simulink model "Q_2_1_PID_with_Anti_Windup"  (R2024b)
settings: Solver=ode45  StartTime=0.0  StopTime=1  FixedStep=0.001  RelTol=1e-3
values from neighbouring files (symbols this model uses):
  delta_c = 1 / sqrt(2)    [PID_calculations.m]    (also in SS_Calculations.m)
  K_D = K_P * T_D    [PID_calculations.m]
  K_I = K_P / T_I    [PID_calculations.m]
  K_P = DeltaK * cos(DeltaPhi)    [PID_calculations.m]
  K_W = 1 / T_W    (= 1485.71428571)    [PID_calculations.m]
  T_L = 5 * w_gc    [PID_calculations.m]
  w_c = 2 * pi * 20    (= 125.663706144)    [PID_calculations.m]    (also in SS_Calculations.m = 314.159265359)
undefined symbols (not defined in the file or in its folder): gbox, rads2rpm, sens
settings Model: Creator=JS  LastModifiedBy=JS

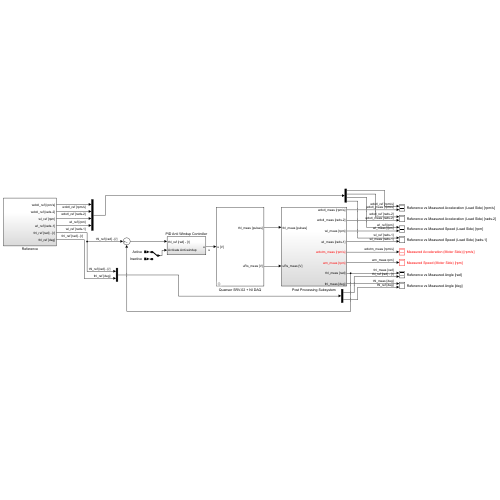
[thumbnail: Simulink's stored preview of the top-level diagram]
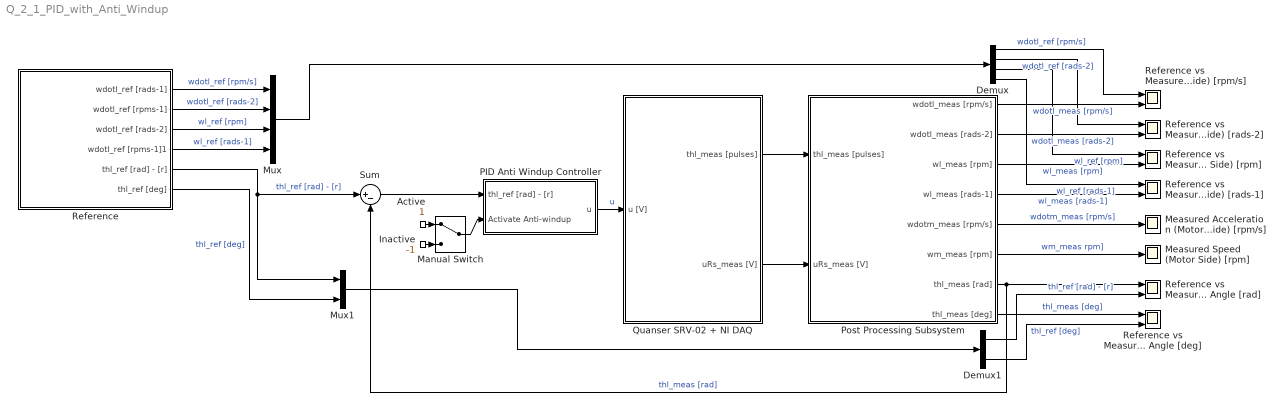
== system Q_2_1_PID_with_Anti_Windup ==
  Active : Constant
  Demux : Demux
  Demux1 : Demux  Outputs=2
  Inactive : Constant  Value=-1
  Manual Switch : ManualSwitch
  Measured Acceleration (Motor Side) [rpm/s] : Scope
  Measured Speed (Motor Side) [rpm] : Scope
  Mux : Mux
  Mux1 : Mux  Inputs=2
  PID Anti Windup Controller : Subsystem
  Post Processing Subsystem : Subsystem
  Quanser SRV-02 + NI DAQ : Subsystem  mask(Quanser SRV-02 (with inertial load) + NI DAQ){Ts=0.001, fricType=Coulomb + viscous}
      mask prompts: Ts "NI DAQ Sample Time:"; fricType "Friction model"
      mask help: Quanser SRV-02 (with inertial load) + NI DAQ model.
      mask init:
      | %%  Sensors data
      | 
      | %   shunt resistor
      | sens.curr.Rs = 0.5;                         %   resistance [Ohm]   
      | sens.curr.uRs_std = 0.01;                   %   voltage noise standard dev [V]                           
      | sens.curr.uRs_var = sens.curr.uRs_std^2;	%   voltage noise variance [V^2]
      | 
      | %   Hewlett-Packard HEDS-5540#A06 optical encoder
      | sens.enc.ppr = 500*4;                       %   pulses per rotation
      | sens.enc.pulse2deg = 360/sens.enc.ppr;      %   [pulses] -> [deg]
      | sens.enc.pulse2rad = 2*pi/sens.enc.ppr;     %   [pulses] -> [rad]
      | sens.enc.deg2pulse = sens.enc.ppr/360;      %   [deg] -> [pulses]
      | sens.enc.rad2pulse = sens.enc.ppr/2/pi;     %   [rad] -> [pulses]
      | 
      | 
      | %%  Data acquisition board (daq) data
      | 
      | %   NI PCI-6221 DAC data
      | daq.dac.bits = 16;                                  %   resolution (bits)
      | daq.dac.fs   = 10;                                  %   full scale 
      | daq.dac.q    = 2*daq.dac.fs/(2^daq.dac.bits-1);     %	quantization
      | 
      | %   NI PCI-6221 ADC data
      | daq.adc.bits = 16;                                  %   resolution (bits)
      | daq.adc.fs   = 10;                                  %   full scale (as set in SLDRT Analog Input block)
      | daq.adc.q    = 2*daq.adc.fs/(2^daq.adc.bits-1);     %   quantization
      mask Help:
      | Riccardo Antonello (antonello@dei.unipd.it)
      | 
      | April 24, 2020
      | 
      | Dept. of Information Engineering, University of Padova
      mask TypeOptions fricType: Coulomb + viscous | Karnopp
  Reference : Subsystem
  Reference vs Measured Acceleration (Load Side) [rads-2] : Scope  NumInputPorts=2
  Reference vs Measured Acceleration (Load Side) [rpm/s] : Scope  NumInputPorts=2
  "Reference vs Measured Angle [deg] " : Scope  NumInputPorts=2
  "Reference vs Measured Angle [rad] " : Scope  NumInputPorts=2
  Reference vs Measured Speed (Load Side) [rads-1] : Scope  NumInputPorts=2
  Reference vs Measured Speed (Load Side) [rpm] : Scope  NumInputPorts=2
  Sum : Sum  Inputs=|+-
  wires:
  Reference/5(thl_ref [rad] - [r]) -> Sum/1, Mux1/1  "thl_ref [rad] - [r]"
  Reference/2(wdotl_ref [rpms-1]) -> Mux/2  "wdotl_ref [rads-2]"
  Reference/1(wdotl_ref [rads-1]) -> Mux/1  "wdotl_ref [rpm/s]"
  Reference/6(thl_ref [deg]) -> Mux1/2  "thl_ref [deg]"
  PID Anti Windup Controller/1(u) -> Quanser SRV-02 + NI DAQ/1(u [V])  "u"
  Quanser SRV-02 + NI DAQ/1(thl_meas [pulses]) -> Post Processing Subsystem/1(thl_meas [pulses])
  Quanser SRV-02 + NI DAQ/2(uRs_meas [V]) -> Post Processing Subsystem/2(uRs_meas [V])
  Post Processing Subsystem/1(wdotl_meas [rpm/s]) -> Reference vs Measured Acceleration (Load Side) [rpm/s]/2  "wdotl_meas [rpm/s]"
  Post Processing Subsystem/8(thl_meas [deg]) -> "Reference vs Measured Angle [deg] "/1  "thl_meas [deg]"
  Post Processing Subsystem/7(thl_meas [rad]) -> "Reference vs Measured Angle [rad] "/1, Sum/2  "thl_meas [rad]"
  Post Processing Subsystem/2(wdotl_meas [rads-2]) -> Reference vs Measured Acceleration (Load Side) [rads-2]/2  "wdotl_meas [rads-2]"
  Post Processing Subsystem/5(wdotm_meas [rpm/s]) -> Measured Acceleration (Motor Side) [rpm/s]/1  "wdotm_meas [rpm/s]"
  Post Processing Subsystem/6(wm_meas [rpm]) -> Measured Speed (Motor Side) [rpm]/1  "wm_meas rpm]"
  Post Processing Subsystem/4(wl_meas [rads-1]) -> Reference vs Measured Speed (Load Side) [rads-1]/2  "wl_meas [rads-1]"
  Post Processing Subsystem/3(wl_meas [rpm]) -> Reference vs Measured Speed (Load Side) [rpm]/2  "wl_meas [rpm]"
  Reference/3(wdotl_ref [rads-2]) -> Mux/3  "wl_ref [rpm]"
  Reference/4(wdotl_ref [rpms-1]1) -> Mux/4  "wl_ref [rads-1]"
  Demux/1 -> Reference vs Measured Acceleration (Load Side) [rpm/s]/1  "wdotl_ref [rpm/s]"
  Demux/2 -> Reference vs Measured Acceleration (Load Side) [rads-2]/1  "wdotl_ref [rads-2]"
  Demux/3 -> Reference vs Measured Speed (Load Side) [rpm]/1  "wl_ref [rpm]"
  Demux/4 -> Reference vs Measured Speed (Load Side) [rads-1]/1  "wl_ref [rads-1]"
  Mux/1 -> Demux/1
  Mux1/1 -> Demux1/1
  Demux1/1 -> "Reference vs Measured Angle [rad] "/2  "thl_ref [rad] - [r]"
  Demux1/2 -> "Reference vs Measured Angle [deg] "/2  "thl_ref [deg]"
  Inactive/1 -> Manual Switch/2
  Active/1 -> Manual Switch/1
  Manual Switch/1 -> PID Anti Windup Controller/2(Activate Anti-windup)
  Sum/1 -> PID Anti Windup Controller/1(thl_ref [rad] - [r])

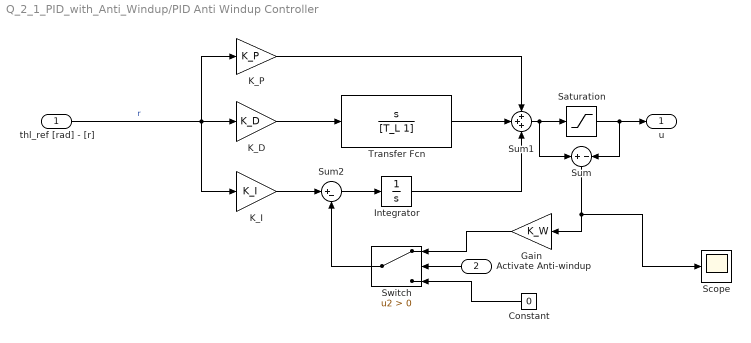
== system Q_2_1_PID_with_Anti_Windup/PID Anti Windup Controller ==
  thl_ref [rad] - [r] : Inport
  Activate Anti-windup : Inport  Port=2
  Constant : Constant  Value=0
  Gain : Gain  Gain=K_W
  Integrator : Integrator  ZeroCross=off
  K_D : Gain  Gain=K_D
  K_I : Gain  Gain=K_I
  K_P : Gain  Gain=K_P
  Saturation : Saturate  UpperLimit=10  LowerLimit=-10  LinearizeAsGain=off
  Scope : Scope
  Sum : Sum  Inputs=+|-
  Sum1 : Sum  Inputs=+++
  Sum2 : Sum  Inputs=|+-
  Switch : Switch  Criteria=u2 > Threshold  SaturateOnIntegerOverflow=off  InputSameDT=off
  Transfer Fcn : TransferFcn  Numerator=[1 0]  Denominator=[T_L 1]
  u : Outport
  wires:
  thl_ref [rad] - [r]/1 -> K_I/1, K_D/1, K_P/1  "r"
  Saturation/1 -> Sum/2, u/1
  Sum1/1 -> Saturation/1, Sum/1
  Transfer Fcn/1 -> Sum1/2
  Integrator/1 -> Sum1/3
  K_P/1 -> Sum1/1
  Activate Anti-windup/1 -> Switch/2
  Gain/1 -> Switch/1
  Constant/1 -> Switch/3
  Sum/1 -> Scope/1, Gain/1
  Switch/1 -> Sum2/2
  K_D/1 -> Transfer Fcn/1
  K_I/1 -> Sum2/1
  Sum2/1 -> Integrator/1

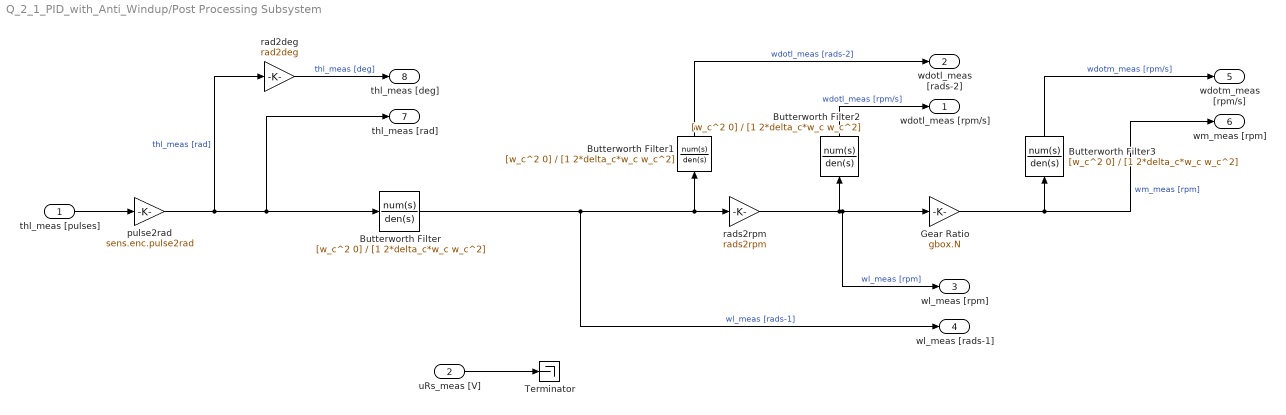
== system Q_2_1_PID_with_Anti_Windup/Post Processing Subsystem ==
  thl_meas [pulses] : Inport
  uRs_meas [V] : Inport  Port=2
  Butterworth Filter{,1..3} (4 alike) : TransferFcn  Numerator=[w_c^2 0]  Denominator=[1 2*delta_c*w_c w_c^2]
  Gear Ratio : Gain  Gain=gbox.N
  Terminator : Terminator
  pulse2rad : Gain  Gain=sens.enc.pulse2rad
  rad2deg : Gain  Gain=rad2deg
  rads2rpm : Gain  Gain=rads2rpm
  wdotl_meas [rpm/s] : Outport
  wdotl_meas [rads-2] : Outport  Port=2
  wl_meas [rpm] : Outport  Port=3
  wl_meas [rads-1] : Outport  Port=4
  wdotm_meas [rpm/s] : Outport  Port=5
  wm_meas [rpm] : Outport  Port=6
  thl_meas [rad] : Outport  Port=7
  thl_meas [deg] : Outport  Port=8
  wires:
  pulse2rad/1 -> Butterworth Filter/1, thl_meas [rad]/1, rad2deg/1  "thl_meas [rad]"
  rad2deg/1 -> thl_meas [deg]/1  "thl_meas [deg]"
  uRs_meas [V]/1 -> Terminator/1
  thl_meas [pulses]/1 -> pulse2rad/1
  Butterworth Filter3/1 -> wdotm_meas [rpm/s]/1  "wdotm_meas [rpm/s]"
  Butterworth Filter2/1 -> wdotl_meas [rpm/s]/1  "wdotl_meas [rpm/s]"
  rads2rpm/1 -> Gear Ratio/1, wl_meas [rpm]/1, Butterworth Filter2/1  "wl_meas [rpm]"
  Butterworth Filter1/1 -> wdotl_meas [rads-2]/1  "wdotl_meas [rads-2]"
  Gear Ratio/1 -> wm_meas [rpm]/1, Butterworth Filter3/1  "wm_meas [rpm]"
  Butterworth Filter/1 -> Butterworth Filter1/1, rads2rpm/1, wl_meas [rads-1]/1  "wl_meas [rads-1]"

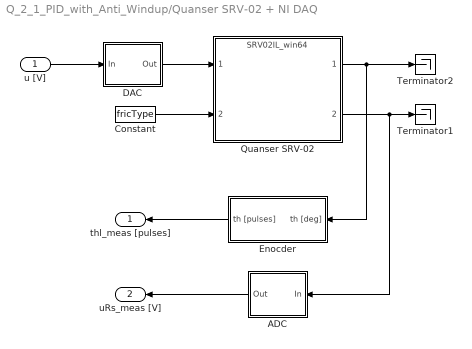
== system Q_2_1_PID_with_Anti_Windup/Quanser SRV-02 + NI DAQ ==
  u [V] : Inport
  ADC : Subsystem
  Constant : Constant  Value=fricType
  DAC : Subsystem
  Enocder : Subsystem
  Quanser SRV-02 : ModelReference  ModelNameDialog=SRV02IL_win64.slxp  ModelReferenceVersion=1.44  CopyOfModelProtected=on
  Terminator1 : Terminator
  Terminator2 : Terminator
  thl_meas [pulses] : Outport
  uRs_meas [V] : Outport  Port=2
  wires:
  Enocder/1(th [pulses]) -> thl_meas [pulses]/1
  ADC/1(Out) -> uRs_meas [V]/1
  DAC/1(Out) -> Quanser SRV-02/1
  Quanser SRV-02/2 -> ADC/1(In), Terminator1/1
  u [V]/1 -> DAC/1(In)
  Quanser SRV-02/1 -> Enocder/1(th [deg]), Terminator2/1
  Constant/1 -> Quanser SRV-02/2

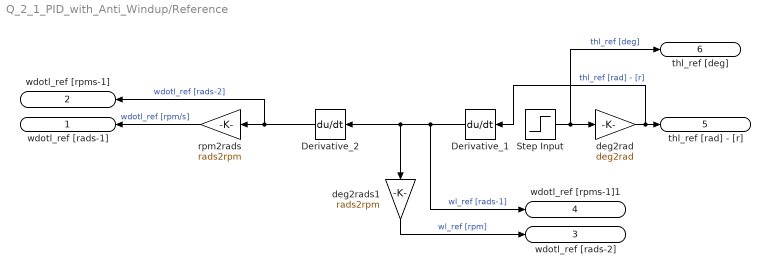
== system Q_2_1_PID_with_Anti_Windup/Reference ==
  Derivative_1 : Derivative
  Derivative_2 : Derivative
  Step Input : Step  Time=0  After=70  SampleTime=0
  deg2rad : Gain  Gain=deg2rad
  deg2rads1 : Gain  Gain=rads2rpm
  rpm2rads : Gain  Gain=rads2rpm
  wdotl_ref [rads-1] : Outport
  wdotl_ref [rpms-1] : Outport  Port=2
  wdotl_ref [rads-2] : Outport  Port=3
  wdotl_ref [rpms-1]1 : Outport  Port=4
  thl_ref [rad] - [r] : Outport  Port=5
  thl_ref [deg] : Outport  Port=6
  wires:
  deg2rad/1 -> Derivative_1/1, thl_ref [rad] - [r]/1  "thl_ref [rad] - [r]"
  Step Input/1 -> thl_ref [deg]/1, deg2rad/1  "thl_ref [deg]"
  Derivative_2/1 -> rpm2rads/1, wdotl_ref [rpms-1]/1  "wdotl_ref [rads-2]"
  rpm2rads/1 -> wdotl_ref [rads-1]/1  "wdotl_ref [rpm/s]"
  Derivative_1/1 -> Derivative_2/1, deg2rads1/1, wdotl_ref [rpms-1]1/1  "wl_ref [rads-1]"
  deg2rads1/1 -> wdotl_ref [rads-2]/1  "wl_ref [rpm]"

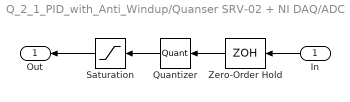
== system Q_2_1_PID_with_Anti_Windup/Quanser SRV-02 + NI DAQ/ADC ==
  In : Inport
  Quantizer : Quantizer  QuantizationInterval=daq.adc.q
  Saturation : Saturate  UpperLimit=daq.adc.fs  LowerLimit=-daq.adc.fs
  Zero-Order Hold : ZeroOrderHold  SampleTime=Ts
  Out : Outport
  wires:
  Saturation/1 -> Out/1
  In/1 -> Zero-Order Hold/1
  Quantizer/1 -> Saturation/1
  Zero-Order Hold/1 -> Quantizer/1

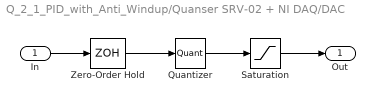
== system Q_2_1_PID_with_Anti_Windup/Quanser SRV-02 + NI DAQ/DAC ==
  In : Inport
  Quantizer : Quantizer  QuantizationInterval=daq.dac.q
  Saturation : Saturate  UpperLimit=daq.dac.fs  LowerLimit=-daq.dac.fs
  Zero-Order Hold : ZeroOrderHold  SampleTime=Ts
  Out : Outport
  wires:
  Quantizer/1 -> Saturation/1
  In/1 -> Zero-Order Hold/1
  Zero-Order Hold/1 -> Quantizer/1
  Saturation/1 -> Out/1

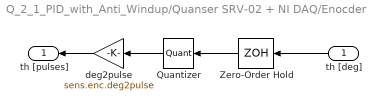
== system Q_2_1_PID_with_Anti_Windup/Quanser SRV-02 + NI DAQ/Enocder ==
  th [deg] : Inport
  Quantizer : Quantizer  QuantizationInterval=sens.enc.pulse2deg
  Zero-Order Hold : ZeroOrderHold  SampleTime=Ts
  deg2pulse : Gain  Gain=sens.enc.deg2pulse
  th [pulses] : Outport
  wires:
  Quantizer/1 -> deg2pulse/1
  th [deg]/1 -> Zero-Order Hold/1
  Zero-Order Hold/1 -> Quantizer/1
  deg2pulse/1 -> th [pulses]/1
